simulink subsystem "Scaling"  (R2024b)
settings: Solver=VariableStepAuto  StartTime=0.0  StopTime=10.0  RelTol=1e-3
undefined symbols (not defined in the file): ADCOffsetVoltageAC, ADCOffsetVoltageDCn, ADCScaleCurrent, ADCScaleVoltageAC, ADCScaleVoltageDCn, ADCScaleVoltageDCp
settings Model: DataDictionary=RectData.sldd  EnableAccessToBaseWorkspace=off  Creator=sgade  LastModifiedBy=sgade

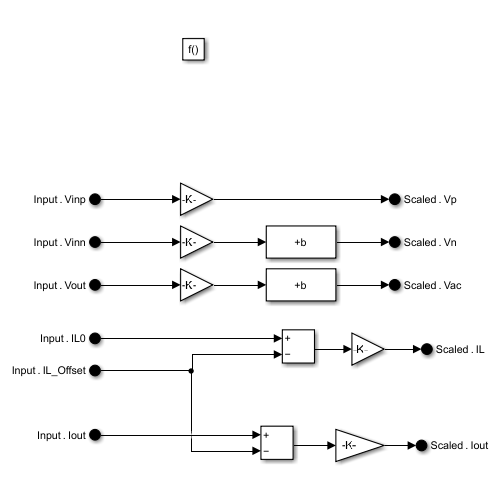
[thumbnail: Simulink's stored preview of the top-level diagram]
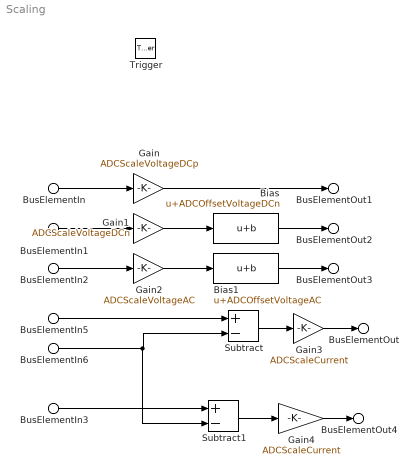
== system Scaling ==
  BusElementIn : Inport  Description=ADCA0  PortName=Input  Element=Vinp
  BusElementIn1 : Inport  Description=ADCA1  PortName=Input  Element=Vinn
  BusElementIn2 : Inport  Description=ADCA2  PortName=Input  Element=Vout
  BusElementIn3 : Inport  Description=ADCA5  PortName=Input  Element=Iout
  BusElementIn5 : Inport  Description=ADCC0  PortName=Input  Element=IL0
  BusElementIn6 : Inport  Description=ADCC1  PortName=Input  Element=IL_Offset
  Trigger : TriggerPort  TriggerType=function-call  VariantControl=(inherit)  PortDimensions=1
  Bias : Bias  Bias=ADCOffsetVoltageDCn  SaturateOnIntegerOverflow=off
  Bias1 : Bias  Bias=ADCOffsetVoltageAC  SaturateOnIntegerOverflow=off
  Gain : Gain  Gain=ADCScaleVoltageDCp
  Gain1 : Gain  Gain=ADCScaleVoltageDCn
  Gain2 : Gain  Gain=ADCScaleVoltageAC
  Gain3 : Gain  Gain=ADCScaleCurrent
  Gain4 : Gain  Gain=ADCScaleCurrent
  Subtract : Sum  Inputs=+-
  Subtract1 : Sum  Inputs=+-
  BusElementOut : Outport  PortName=Scaled  Element=IL
  BusElementOut1 : Outport  PortName=Scaled  Element=Vp
  BusElementOut2 : Outport  PortName=Scaled  Element=Vn
  BusElementOut3 : Outport  PortName=Scaled  Element=Vac
  BusElementOut4 : Outport  PortName=Scaled  Element=Iout
  wires:
  BusElementIn/1 -> Gain/1
  Gain/1 -> BusElementOut1/1
  BusElementIn1/1 -> Gain1/1
  Gain1/1 -> Bias/1
  BusElementIn2/1 -> Gain2/1
  Gain2/1 -> Bias1/1
  Bias/1 -> BusElementOut2/1
  Bias1/1 -> BusElementOut3/1
  BusElementIn5/1 -> Subtract/1
  BusElementIn6/1 -> Subtract1/2, Subtract/2
  Subtract/1 -> Gain3/1
  Gain3/1 -> BusElementOut/1
  Gain4/1 -> BusElementOut4/1
  Subtract1/1 -> Gain4/1
  BusElementIn3/1 -> Subtract1/1
